simulink model "Crane_rigid"  (R2021b)
settings: Solver=ode15s  StartTime=0.0  StopTime=t_f  MaxStep=max_step_size  RelTol=1e-3
values from neighbouring files (symbols this model uses):
  a_d_full_y = circshift(a_d_full_x,floor(1/h))/2    [modify_tracking.m]
  cont_param_10 = in    [double_pendulum.m]    (also in optimize_10_SMC_single_first_explicit.m = cont_param_10_surrogateopt)
  cont_param_11 = in    [double_pendulum.m]    (also in optimize_11_SMC_single_first_implicit.m = cont_param_11_surrogateopt)
  cont_param_12 = in    [double_pendulum.m]    (also in optimize_12_SMC_single_last_explicit.m = cont_param_12_surrogateopt)
  cont_param_13 = in    [double_pendulum.m]    (also in optimize_13_SMC_single_last_implicit.m = cont_param_13_surrogateopt)
  cont_param_14 = in    [double_pendulum.m]    (also in optimize_14_SMC_double_explicit.m = cont_param_14_surrogateopt)
  cont_param_15 = in    [double_pendulum.m]    (also in optimize_15_SMC_double_implicit.m = cont_param_15_surrogateopt)
  cont_param_16 = in    [double_pendulum.m]
  cont_param_17 = in    [double_pendulum.m]
  cont_param_18 = in    [double_pendulum.m]
  cont_param_19 = in    [double_pendulum.m]
  cont_param_4 = in    [double_pendulum.m]
  cont_param_5 = in    [double_pendulum.m]
  cont_param_6 = in    [double_pendulum.m]
  cont_param_7 = in    [double_pendulum.m]
  cont_param_8 = in    [double_pendulum.m]
  cont_param_9 = in    [double_pendulum.m]
  h = 1e-5    (= 1e-05)    [Conference_paper.m]    (also in Latest.m)
  m = 10    [Conference_paper.m]    (also in Latest.m = 100; control_8_collocated_PD_tracking.m = load_mass+hook_mass+cable_mass_total)
  method_select = Method    [main_run.m]    (also in modify_tracking.m = 3)
  N = floor(t_f / h)    [control_2_zero_vibration.m]    (also in control_3_ZVD.m; modify_tracking.m = 3)
  s = c1*(x-xd)+c2*(v-vd)+c3*theta_dot_1+c4*theta_1    [control_10_SMC_single_first_explicit.m]    (also in control_11_SMC_single_first_implicit.m = c1*(x-xd)+c2*(v-vd)+c3*theta_dot+c4*theta; control_12_SMC_single_last_explicit.m = c1*(x-xd)+c2*(v-vd)+c3*theta_dot_2+c4*theta_2; control_13_SMC_single_last_implicit.m = c1*(x-xd)+c2*(v-vd)+c3*theta_dot+c4*theta; control_14_SMC_double_explicit.m = (v-vd)+lambda*(x-xd)+alpha*theta_1+beta*theta_2)
  sin_traj_w = 0.5    [modify_tracking.m]
  X = ex+lambda*sin(theta)    [control_16_PD_energy_first.m]    (also in control_17_PD_energy_last.m)
  Z = cont_param_8(4)    [control_8_collocated_PD_tracking.m]
undefined symbols (not defined in the file or in its folder): a_d_full_x, all_initial_sway, c_actuator, cable_length, cable_mass_total, cart_disturbance_amp, cart_mass, delay_time, first_link_sway, hook_mass, last_piece_length, load_disturbance_amp, number_of_pendulums, payload_mass, sat_const, sin_traj_A, t_f, total_mass, traj_number, unbalanced_factor, Y
libraries: nesl_utility x180, sm_lib x138, commchan3 x8
(part 3 of 3)

== system Crane_rigid/All pendulum/Angle sensor 2 ==
  Gain : Gain  Gain=-1
  Gain1 : Gain  Gain=-1
  PS-Simulink Converter{,1..7} (8 alike) : nesl_utility/PS-Simulink Converter  PhysicalDomain=network_engine_domain  SubClassName=ps_output  LeftPortType=input  RightPortType=output  PseudoPeriodic=off  Frequencies=[]  Unit=inherit  AffineConversion=off
      settings: SourceProductBaseCode=PW,SS
  Product : Product  Inputs=*/
  Product1 : Product  Inputs=*/
  Sin1 : Trigonometry  Operator=atan
  Sin2 : Trigonometry  Operator=atan
  Sum{,1..3} (4 alike) : Sum  Inputs=|+-
  Transform Sensor1 : sm_lib/Frames and Transforms/Transform Sensor  MeasurementFrame=World  SenseAngle=off  SenseAxis=off  SenseAngle1=off  SenseAngle2=off  SenseAngle3=off  SenseQ=off  SenseR=off  SenseOmegaX=off  SenseOmegaY=off  SenseOmegaZ=off  SenseOmega1=off  SenseOmega2=off  SenseOmega3=off  SenseQDot=off  SenseRDot=off  SenseAlphaX=off  SenseAlphaY=off  SenseAlphaZ=off  SenseAlpha1=off  SenseAlpha2=off  SenseAlpha3=off  SenseQDDot=off  SenseRDDot=off  SenseX=on  SenseY=on  SenseZ=on  SenseRad=off  SenseAzim=off  SenseDist=off  SenseInc=off  SenseXDot=off  SenseYDot=off  SenseZDot=off  SenseRadDot=off  SenseAzimDot=off  SenseDistDot=off  SenseIncDot=off  SenseXDDot=off  SenseYDDot=off  SenseZDDot=off  SenseRadDDot=off  SenseAzimDDot=off  SenseDistDDot=off  SenseIncDDot=off
  Transform Sensor2 : sm_lib/Frames and Transforms/Transform Sensor  MeasurementFrame=World  SenseAngle=off  SenseAxis=off  SenseAngle1=off  SenseAngle2=off  SenseAngle3=off  SenseQ=off  SenseR=off  SenseOmegaX=off  SenseOmegaY=off  SenseOmegaZ=off  SenseOmega1=off  SenseOmega2=off  SenseOmega3=off  SenseQDot=off  SenseRDot=off  SenseAlphaX=off  SenseAlphaY=off  SenseAlphaZ=off  SenseAlpha1=off  SenseAlpha2=off  SenseAlpha3=off  SenseQDDot=off  SenseRDDot=off  SenseX=on  SenseY=on  SenseZ=on  SenseRad=off  SenseAzim=off  SenseDist=off  SenseInc=off  SenseXDot=off  SenseYDot=off  SenseZDot=off  SenseRadDot=off  SenseAzimDot=off  SenseDistDot=off  SenseIncDot=off  SenseXDDot=off  SenseYDDot=off  SenseZDDot=off  SenseRadDDot=off  SenseAzimDDot=off  SenseDistDDot=off  SenseIncDDot=off
  World Frame : sm_lib/Frames and Transforms/World Frame
  Con1_up : PMIOPort  Side=Left
  Con2_down : PMIOPort  Port=2  Side=Left
  Angle_x : Outport
  Angle_y : Outport  Port=2
  wires:
  Sin1/1 -> Angle_y/1
  Sin2/1 -> Angle_x/1
  Sum/1 -> Gain/1
  Gain1/1 -> Product1/1
  Sum3/1 -> Product1/2
  Sum2/1 -> Gain1/1
  Product1/1 -> Sin1/1
  PS-Simulink Converter6/1 -> Sum3/1
  PS-Simulink Converter1/1 -> Sum/2
  PS-Simulink Converter5/1 -> Sum2/2
  PS-Simulink Converter4/1 -> Sum2/1
  PS-Simulink Converter7/1 -> Sum3/2
  Gain/1 -> Product/1
  PS-Simulink Converter3/1 -> Sum1/2
  PS-Simulink Converter2/1 -> Sum1/1
  Product/1 -> Sin2/1
  Sum1/1 -> Product/2
  PS-Simulink Converter/1 -> Sum/1
  connections:
  Con2_down/RConn1 -- Transform Sensor2/RConn1
  Transform Sensor1/RConn1 -- Con1_up/RConn1
  PS-Simulink Converter/LConn1 -- Transform Sensor1/RConn2
  Transform Sensor2/RConn2 -- PS-Simulink Converter1/LConn1
  PS-Simulink Converter4/LConn1 -- Transform Sensor1/RConn3
  PS-Simulink Converter5/LConn1 -- Transform Sensor2/RConn3
  PS-Simulink Converter2/LConn1 -- PS-Simulink Converter6/LConn1 -- Transform Sensor1/RConn4
  PS-Simulink Converter3/LConn1 -- PS-Simulink Converter7/LConn1 -- Transform Sensor2/RConn4
  Transform Sensor1/LConn1 -- Transform Sensor2/LConn1 -- World Frame/RConn1

== system Crane_rigid/All pendulum/Angle sensor 20 ==
  Gain : Gain  Gain=-1
  Gain1 : Gain  Gain=-1
  PS-Simulink Converter{,1..7} (8 alike) : nesl_utility/PS-Simulink Converter  PhysicalDomain=network_engine_domain  SubClassName=ps_output  LeftPortType=input  RightPortType=output  PseudoPeriodic=off  Frequencies=[]  Unit=inherit  AffineConversion=off
      settings: SourceProductBaseCode=PW,SS
  Product : Product  Inputs=*/
  Product1 : Product  Inputs=*/
  Sin1 : Trigonometry  Operator=atan
  Sin2 : Trigonometry  Operator=atan
  Sum{,1..3} (4 alike) : Sum  Inputs=|+-
  Transform Sensor1 : sm_lib/Frames and Transforms/Transform Sensor  MeasurementFrame=World  SenseAngle=off  SenseAxis=off  SenseAngle1=off  SenseAngle2=off  SenseAngle3=off  SenseQ=off  SenseR=off  SenseOmegaX=off  SenseOmegaY=off  SenseOmegaZ=off  SenseOmega1=off  SenseOmega2=off  SenseOmega3=off  SenseQDot=off  SenseRDot=off  SenseAlphaX=off  SenseAlphaY=off  SenseAlphaZ=off  SenseAlpha1=off  SenseAlpha2=off  SenseAlpha3=off  SenseQDDot=off  SenseRDDot=off  SenseX=on  SenseY=on  SenseZ=on  SenseRad=off  SenseAzim=off  SenseDist=off  SenseInc=off  SenseXDot=off  SenseYDot=off  SenseZDot=off  SenseRadDot=off  SenseAzimDot=off  SenseDistDot=off  SenseIncDot=off  SenseXDDot=off  SenseYDDot=off  SenseZDDot=off  SenseRadDDot=off  SenseAzimDDot=off  SenseDistDDot=off  SenseIncDDot=off
  Transform Sensor2 : sm_lib/Frames and Transforms/Transform Sensor  MeasurementFrame=World  SenseAngle=off  SenseAxis=off  SenseAngle1=off  SenseAngle2=off  SenseAngle3=off  SenseQ=off  SenseR=off  SenseOmegaX=off  SenseOmegaY=off  SenseOmegaZ=off  SenseOmega1=off  SenseOmega2=off  SenseOmega3=off  SenseQDot=off  SenseRDot=off  SenseAlphaX=off  SenseAlphaY=off  SenseAlphaZ=off  SenseAlpha1=off  SenseAlpha2=off  SenseAlpha3=off  SenseQDDot=off  SenseRDDot=off  SenseX=on  SenseY=on  SenseZ=on  SenseRad=off  SenseAzim=off  SenseDist=off  SenseInc=off  SenseXDot=off  SenseYDot=off  SenseZDot=off  SenseRadDot=off  SenseAzimDot=off  SenseDistDot=off  SenseIncDot=off  SenseXDDot=off  SenseYDDot=off  SenseZDDot=off  SenseRadDDot=off  SenseAzimDDot=off  SenseDistDDot=off  SenseIncDDot=off
  World Frame : sm_lib/Frames and Transforms/World Frame
  Con1_up : PMIOPort  Side=Left
  Con2_down : PMIOPort  Port=2  Side=Left
  Angle_x : Outport
  Angle_y : Outport  Port=2
  wires:
  Sin1/1 -> Angle_y/1
  Sin2/1 -> Angle_x/1
  Sum/1 -> Gain/1
  Gain1/1 -> Product1/1
  Sum3/1 -> Product1/2
  Sum2/1 -> Gain1/1
  Product1/1 -> Sin1/1
  PS-Simulink Converter6/1 -> Sum3/1
  PS-Simulink Converter1/1 -> Sum/2
  PS-Simulink Converter5/1 -> Sum2/2
  PS-Simulink Converter4/1 -> Sum2/1
  PS-Simulink Converter7/1 -> Sum3/2
  Gain/1 -> Product/1
  PS-Simulink Converter3/1 -> Sum1/2
  PS-Simulink Converter2/1 -> Sum1/1
  Product/1 -> Sin2/1
  Sum1/1 -> Product/2
  PS-Simulink Converter/1 -> Sum/1
  connections:
  Con2_down/RConn1 -- Transform Sensor2/RConn1
  Transform Sensor1/RConn1 -- Con1_up/RConn1
  PS-Simulink Converter/LConn1 -- Transform Sensor1/RConn2
  Transform Sensor2/RConn2 -- PS-Simulink Converter1/LConn1
  PS-Simulink Converter4/LConn1 -- Transform Sensor1/RConn3
  PS-Simulink Converter5/LConn1 -- Transform Sensor2/RConn3
  PS-Simulink Converter2/LConn1 -- PS-Simulink Converter6/LConn1 -- Transform Sensor1/RConn4
  PS-Simulink Converter3/LConn1 -- PS-Simulink Converter7/LConn1 -- Transform Sensor2/RConn4
  Transform Sensor1/LConn1 -- Transform Sensor2/LConn1 -- World Frame/RConn1

== system Crane_rigid/All pendulum/Angle sensor 21 ==
  Gain : Gain  Gain=-1
  Gain1 : Gain  Gain=-1
  PS-Simulink Converter{,1..7} (8 alike) : nesl_utility/PS-Simulink Converter  PhysicalDomain=network_engine_domain  SubClassName=ps_output  LeftPortType=input  RightPortType=output  PseudoPeriodic=off  Frequencies=[]  Unit=inherit  AffineConversion=off
      settings: SourceProductBaseCode=PW,SS
  Product : Product  Inputs=*/
  Product1 : Product  Inputs=*/
  Sin1 : Trigonometry  Operator=atan
  Sin2 : Trigonometry  Operator=atan
  Sum{,1..3} (4 alike) : Sum  Inputs=|+-
  Transform Sensor1 : sm_lib/Frames and Transforms/Transform Sensor  MeasurementFrame=World  SenseAngle=off  SenseAxis=off  SenseAngle1=off  SenseAngle2=off  SenseAngle3=off  SenseQ=off  SenseR=off  SenseOmegaX=off  SenseOmegaY=off  SenseOmegaZ=off  SenseOmega1=off  SenseOmega2=off  SenseOmega3=off  SenseQDot=off  SenseRDot=off  SenseAlphaX=off  SenseAlphaY=off  SenseAlphaZ=off  SenseAlpha1=off  SenseAlpha2=off  SenseAlpha3=off  SenseQDDot=off  SenseRDDot=off  SenseX=on  SenseY=on  SenseZ=on  SenseRad=off  SenseAzim=off  SenseDist=off  SenseInc=off  SenseXDot=off  SenseYDot=off  SenseZDot=off  SenseRadDot=off  SenseAzimDot=off  SenseDistDot=off  SenseIncDot=off  SenseXDDot=off  SenseYDDot=off  SenseZDDot=off  SenseRadDDot=off  SenseAzimDDot=off  SenseDistDDot=off  SenseIncDDot=off
  Transform Sensor2 : sm_lib/Frames and Transforms/Transform Sensor  MeasurementFrame=World  SenseAngle=off  SenseAxis=off  SenseAngle1=off  SenseAngle2=off  SenseAngle3=off  SenseQ=off  SenseR=off  SenseOmegaX=off  SenseOmegaY=off  SenseOmegaZ=off  SenseOmega1=off  SenseOmega2=off  SenseOmega3=off  SenseQDot=off  SenseRDot=off  SenseAlphaX=off  SenseAlphaY=off  SenseAlphaZ=off  SenseAlpha1=off  SenseAlpha2=off  SenseAlpha3=off  SenseQDDot=off  SenseRDDot=off  SenseX=on  SenseY=on  SenseZ=on  SenseRad=off  SenseAzim=off  SenseDist=off  SenseInc=off  SenseXDot=off  SenseYDot=off  SenseZDot=off  SenseRadDot=off  SenseAzimDot=off  SenseDistDot=off  SenseIncDot=off  SenseXDDot=off  SenseYDDot=off  SenseZDDot=off  SenseRadDDot=off  SenseAzimDDot=off  SenseDistDDot=off  SenseIncDDot=off
  World Frame : sm_lib/Frames and Transforms/World Frame
  Con1_up : PMIOPort  Side=Left
  Con2_down : PMIOPort  Port=2  Side=Left
  Angle_x : Outport
  Angle_y : Outport  Port=2
  wires:
  PS-Simulink Converter/1 -> Sum/1
  Sum1/1 -> Product/2
  Product/1 -> Sin2/1
  PS-Simulink Converter2/1 -> Sum1/1
  PS-Simulink Converter3/1 -> Sum1/2
  Gain/1 -> Product/1
  PS-Simulink Converter7/1 -> Sum3/2
  PS-Simulink Converter4/1 -> Sum2/1
  PS-Simulink Converter5/1 -> Sum2/2
  PS-Simulink Converter1/1 -> Sum/2
  PS-Simulink Converter6/1 -> Sum3/1
  Product1/1 -> Sin1/1
  Sum2/1 -> Gain1/1
  Sum3/1 -> Product1/2
  Gain1/1 -> Product1/1
  Sum/1 -> Gain/1
  Sin2/1 -> Angle_x/1
  Sin1/1 -> Angle_y/1
  connections:
  World Frame/RConn1 -- Transform Sensor2/LConn1 -- Transform Sensor1/LConn1
  Transform Sensor2/RConn4 -- PS-Simulink Converter7/LConn1 -- PS-Simulink Converter3/LConn1
  Transform Sensor1/RConn4 -- PS-Simulink Converter6/LConn1 -- PS-Simulink Converter2/LConn1
  PS-Simulink Converter5/LConn1 -- Transform Sensor2/RConn3
  PS-Simulink Converter4/LConn1 -- Transform Sensor1/RConn3
  Transform Sensor2/RConn2 -- PS-Simulink Converter1/LConn1
  PS-Simulink Converter/LConn1 -- Transform Sensor1/RConn2
  Transform Sensor1/RConn1 -- Con1_up/RConn1
  Con2_down/RConn1 -- Transform Sensor2/RConn1

== system Crane_rigid/All pendulum/Angle sensor 3 ==
  Gain : Gain  Gain=-1
  Gain1 : Gain  Gain=-1
  PS-Simulink Converter{,1..7} (8 alike) : nesl_utility/PS-Simulink Converter  PhysicalDomain=network_engine_domain  SubClassName=ps_output  LeftPortType=input  RightPortType=output  PseudoPeriodic=off  Frequencies=[]  Unit=inherit  AffineConversion=off
      settings: SourceProductBaseCode=PW,SS
  Product : Product  Inputs=*/
  Product1 : Product  Inputs=*/
  Sin1 : Trigonometry  Operator=atan
  Sin2 : Trigonometry  Operator=atan
  Sum{,1..3} (4 alike) : Sum  Inputs=|+-
  Transform Sensor1 : sm_lib/Frames and Transforms/Transform Sensor  MeasurementFrame=World  SenseAngle=off  SenseAxis=off  SenseAngle1=off  SenseAngle2=off  SenseAngle3=off  SenseQ=off  SenseR=off  SenseOmegaX=off  SenseOmegaY=off  SenseOmegaZ=off  SenseOmega1=off  SenseOmega2=off  SenseOmega3=off  SenseQDot=off  SenseRDot=off  SenseAlphaX=off  SenseAlphaY=off  SenseAlphaZ=off  SenseAlpha1=off  SenseAlpha2=off  SenseAlpha3=off  SenseQDDot=off  SenseRDDot=off  SenseX=on  SenseY=on  SenseZ=on  SenseRad=off  SenseAzim=off  SenseDist=off  SenseInc=off  SenseXDot=off  SenseYDot=off  SenseZDot=off  SenseRadDot=off  SenseAzimDot=off  SenseDistDot=off  SenseIncDot=off  SenseXDDot=off  SenseYDDot=off  SenseZDDot=off  SenseRadDDot=off  SenseAzimDDot=off  SenseDistDDot=off  SenseIncDDot=off
  Transform Sensor2 : sm_lib/Frames and Transforms/Transform Sensor  MeasurementFrame=World  SenseAngle=off  SenseAxis=off  SenseAngle1=off  SenseAngle2=off  SenseAngle3=off  SenseQ=off  SenseR=off  SenseOmegaX=off  SenseOmegaY=off  SenseOmegaZ=off  SenseOmega1=off  SenseOmega2=off  SenseOmega3=off  SenseQDot=off  SenseRDot=off  SenseAlphaX=off  SenseAlphaY=off  SenseAlphaZ=off  SenseAlpha1=off  SenseAlpha2=off  SenseAlpha3=off  SenseQDDot=off  SenseRDDot=off  SenseX=on  SenseY=on  SenseZ=on  SenseRad=off  SenseAzim=off  SenseDist=off  SenseInc=off  SenseXDot=off  SenseYDot=off  SenseZDot=off  SenseRadDot=off  SenseAzimDot=off  SenseDistDot=off  SenseIncDot=off  SenseXDDot=off  SenseYDDot=off  SenseZDDot=off  SenseRadDDot=off  SenseAzimDDot=off  SenseDistDDot=off  SenseIncDDot=off
  World Frame : sm_lib/Frames and Transforms/World Frame
  Con1_up : PMIOPort  Side=Left
  Con2_down : PMIOPort  Port=2  Side=Left
  Angle_x : Outport
  Angle_y : Outport  Port=2
  wires:
  Sin1/1 -> Angle_y/1
  Sin2/1 -> Angle_x/1
  Sum/1 -> Gain/1
  Gain1/1 -> Product1/1
  Sum3/1 -> Product1/2
  Sum2/1 -> Gain1/1
  Product1/1 -> Sin1/1
  PS-Simulink Converter6/1 -> Sum3/1
  PS-Simulink Converter1/1 -> Sum/2
  PS-Simulink Converter5/1 -> Sum2/2
  PS-Simulink Converter4/1 -> Sum2/1
  PS-Simulink Converter7/1 -> Sum3/2
  Gain/1 -> Product/1
  PS-Simulink Converter3/1 -> Sum1/2
  PS-Simulink Converter2/1 -> Sum1/1
  Product/1 -> Sin2/1
  Sum1/1 -> Product/2
  PS-Simulink Converter/1 -> Sum/1
  connections:
  Con2_down/RConn1 -- Transform Sensor2/RConn1
  Transform Sensor1/RConn1 -- Con1_up/RConn1
  PS-Simulink Converter/LConn1 -- Transform Sensor1/RConn2
  Transform Sensor2/RConn2 -- PS-Simulink Converter1/LConn1
  PS-Simulink Converter4/LConn1 -- Transform Sensor1/RConn3
  PS-Simulink Converter5/LConn1 -- Transform Sensor2/RConn3
  PS-Simulink Converter2/LConn1 -- PS-Simulink Converter6/LConn1 -- Transform Sensor1/RConn4
  PS-Simulink Converter3/LConn1 -- PS-Simulink Converter7/LConn1 -- Transform Sensor2/RConn4
  Transform Sensor1/LConn1 -- Transform Sensor2/LConn1 -- World Frame/RConn1

== system Crane_rigid/All pendulum/Angle sensor 4 ==
  Gain : Gain  Gain=-1
  Gain1 : Gain  Gain=-1
  PS-Simulink Converter{,1..7} (8 alike) : nesl_utility/PS-Simulink Converter  PhysicalDomain=network_engine_domain  SubClassName=ps_output  LeftPortType=input  RightPortType=output  PseudoPeriodic=off  Frequencies=[]  Unit=inherit  AffineConversion=off
      settings: SourceProductBaseCode=PW,SS
  Product : Product  Inputs=*/
  Product1 : Product  Inputs=*/
  Sin1 : Trigonometry  Operator=atan
  Sin2 : Trigonometry  Operator=atan
  Sum{,1..3} (4 alike) : Sum  Inputs=|+-
  Transform Sensor1 : sm_lib/Frames and Transforms/Transform Sensor  MeasurementFrame=World  SenseAngle=off  SenseAxis=off  SenseAngle1=off  SenseAngle2=off  SenseAngle3=off  SenseQ=off  SenseR=off  SenseOmegaX=off  SenseOmegaY=off  SenseOmegaZ=off  SenseOmega1=off  SenseOmega2=off  SenseOmega3=off  SenseQDot=off  SenseRDot=off  SenseAlphaX=off  SenseAlphaY=off  SenseAlphaZ=off  SenseAlpha1=off  SenseAlpha2=off  SenseAlpha3=off  SenseQDDot=off  SenseRDDot=off  SenseX=on  SenseY=on  SenseZ=on  SenseRad=off  SenseAzim=off  SenseDist=off  SenseInc=off  SenseXDot=off  SenseYDot=off  SenseZDot=off  SenseRadDot=off  SenseAzimDot=off  SenseDistDot=off  SenseIncDot=off  SenseXDDot=off  SenseYDDot=off  SenseZDDot=off  SenseRadDDot=off  SenseAzimDDot=off  SenseDistDDot=off  SenseIncDDot=off
  Transform Sensor2 : sm_lib/Frames and Transforms/Transform Sensor  MeasurementFrame=World  SenseAngle=off  SenseAxis=off  SenseAngle1=off  SenseAngle2=off  SenseAngle3=off  SenseQ=off  SenseR=off  SenseOmegaX=off  SenseOmegaY=off  SenseOmegaZ=off  SenseOmega1=off  SenseOmega2=off  SenseOmega3=off  SenseQDot=off  SenseRDot=off  SenseAlphaX=off  SenseAlphaY=off  SenseAlphaZ=off  SenseAlpha1=off  SenseAlpha2=off  SenseAlpha3=off  SenseQDDot=off  SenseRDDot=off  SenseX=on  SenseY=on  SenseZ=on  SenseRad=off  SenseAzim=off  SenseDist=off  SenseInc=off  SenseXDot=off  SenseYDot=off  SenseZDot=off  SenseRadDot=off  SenseAzimDot=off  SenseDistDot=off  SenseIncDot=off  SenseXDDot=off  SenseYDDot=off  SenseZDDot=off  SenseRadDDot=off  SenseAzimDDot=off  SenseDistDDot=off  SenseIncDDot=off
  World Frame : sm_lib/Frames and Transforms/World Frame
  Con1_up : PMIOPort  Side=Left
  Con2_down : PMIOPort  Port=2  Side=Left
  Angle_x : Outport
  Angle_y : Outport  Port=2
  wires:
  Sin1/1 -> Angle_y/1
  Sin2/1 -> Angle_x/1
  Sum/1 -> Gain/1
  Gain1/1 -> Product1/1
  Sum3/1 -> Product1/2
  Sum2/1 -> Gain1/1
  Product1/1 -> Sin1/1
  PS-Simulink Converter6/1 -> Sum3/1
  PS-Simulink Converter1/1 -> Sum/2
  PS-Simulink Converter5/1 -> Sum2/2
  PS-Simulink Converter4/1 -> Sum2/1
  PS-Simulink Converter7/1 -> Sum3/2
  Gain/1 -> Product/1
  PS-Simulink Converter3/1 -> Sum1/2
  PS-Simulink Converter2/1 -> Sum1/1
  Product/1 -> Sin2/1
  Sum1/1 -> Product/2
  PS-Simulink Converter/1 -> Sum/1
  connections:
  Con2_down/RConn1 -- Transform Sensor2/RConn1
  Transform Sensor1/RConn1 -- Con1_up/RConn1
  PS-Simulink Converter/LConn1 -- Transform Sensor1/RConn2
  Transform Sensor2/RConn2 -- PS-Simulink Converter1/LConn1
  PS-Simulink Converter4/LConn1 -- Transform Sensor1/RConn3
  PS-Simulink Converter5/LConn1 -- Transform Sensor2/RConn3
  PS-Simulink Converter2/LConn1 -- PS-Simulink Converter6/LConn1 -- Transform Sensor1/RConn4
  PS-Simulink Converter3/LConn1 -- PS-Simulink Converter7/LConn1 -- Transform Sensor2/RConn4
  Transform Sensor1/LConn1 -- Transform Sensor2/LConn1 -- World Frame/RConn1

== system Crane_rigid/All pendulum/Angle sensor 5 ==
  Gain : Gain  Gain=-1
  Gain1 : Gain  Gain=-1
  PS-Simulink Converter{,1..7} (8 alike) : nesl_utility/PS-Simulink Converter  PhysicalDomain=network_engine_domain  SubClassName=ps_output  LeftPortType=input  RightPortType=output  PseudoPeriodic=off  Frequencies=[]  Unit=inherit  AffineConversion=off
      settings: SourceProductBaseCode=PW,SS
  Product : Product  Inputs=*/
  Product1 : Product  Inputs=*/
  Sin1 : Trigonometry  Operator=atan
  Sin2 : Trigonometry  Operator=atan
  Sum{,1..3} (4 alike) : Sum  Inputs=|+-
  Transform Sensor1 : sm_lib/Frames and Transforms/Transform Sensor  MeasurementFrame=World  SenseAngle=off  SenseAxis=off  SenseAngle1=off  SenseAngle2=off  SenseAngle3=off  SenseQ=off  SenseR=off  SenseOmegaX=off  SenseOmegaY=off  SenseOmegaZ=off  SenseOmega1=off  SenseOmega2=off  SenseOmega3=off  SenseQDot=off  SenseRDot=off  SenseAlphaX=off  SenseAlphaY=off  SenseAlphaZ=off  SenseAlpha1=off  SenseAlpha2=off  SenseAlpha3=off  SenseQDDot=off  SenseRDDot=off  SenseX=on  SenseY=on  SenseZ=on  SenseRad=off  SenseAzim=off  SenseDist=off  SenseInc=off  SenseXDot=off  SenseYDot=off  SenseZDot=off  SenseRadDot=off  SenseAzimDot=off  SenseDistDot=off  SenseIncDot=off  SenseXDDot=off  SenseYDDot=off  SenseZDDot=off  SenseRadDDot=off  SenseAzimDDot=off  SenseDistDDot=off  SenseIncDDot=off
  Transform Sensor2 : sm_lib/Frames and Transforms/Transform Sensor  MeasurementFrame=World  SenseAngle=off  SenseAxis=off  SenseAngle1=off  SenseAngle2=off  SenseAngle3=off  SenseQ=off  SenseR=off  SenseOmegaX=off  SenseOmegaY=off  SenseOmegaZ=off  SenseOmega1=off  SenseOmega2=off  SenseOmega3=off  SenseQDot=off  SenseRDot=off  SenseAlphaX=off  SenseAlphaY=off  SenseAlphaZ=off  SenseAlpha1=off  SenseAlpha2=off  SenseAlpha3=off  SenseQDDot=off  SenseRDDot=off  SenseX=on  SenseY=on  SenseZ=on  SenseRad=off  SenseAzim=off  SenseDist=off  SenseInc=off  SenseXDot=off  SenseYDot=off  SenseZDot=off  SenseRadDot=off  SenseAzimDot=off  SenseDistDot=off  SenseIncDot=off  SenseXDDot=off  SenseYDDot=off  SenseZDDot=off  SenseRadDDot=off  SenseAzimDDot=off  SenseDistDDot=off  SenseIncDDot=off
  World Frame : sm_lib/Frames and Transforms/World Frame
  Con1_up : PMIOPort  Side=Left
  Con2_down : PMIOPort  Port=2  Side=Left
  Angle_x : Outport
  Angle_y : Outport  Port=2
  wires:
  PS-Simulink Converter/1 -> Sum/1
  Sum1/1 -> Product/2
  Product/1 -> Sin2/1
  PS-Simulink Converter2/1 -> Sum1/1
  PS-Simulink Converter3/1 -> Sum1/2
  Gain/1 -> Product/1
  PS-Simulink Converter7/1 -> Sum3/2
  PS-Simulink Converter4/1 -> Sum2/1
  PS-Simulink Converter5/1 -> Sum2/2
  PS-Simulink Converter1/1 -> Sum/2
  PS-Simulink Converter6/1 -> Sum3/1
  Product1/1 -> Sin1/1
  Sum2/1 -> Gain1/1
  Sum3/1 -> Product1/2
  Gain1/1 -> Product1/1
  Sum/1 -> Gain/1
  Sin2/1 -> Angle_x/1
  Sin1/1 -> Angle_y/1
  connections:
  World Frame/RConn1 -- Transform Sensor2/LConn1 -- Transform Sensor1/LConn1
  Transform Sensor2/RConn4 -- PS-Simulink Converter7/LConn1 -- PS-Simulink Converter3/LConn1
  Transform Sensor1/RConn4 -- PS-Simulink Converter6/LConn1 -- PS-Simulink Converter2/LConn1
  PS-Simulink Converter5/LConn1 -- Transform Sensor2/RConn3
  PS-Simulink Converter4/LConn1 -- Transform Sensor1/RConn3
  Transform Sensor2/RConn2 -- PS-Simulink Converter1/LConn1
  PS-Simulink Converter/LConn1 -- Transform Sensor1/RConn2
  Transform Sensor1/RConn1 -- Con1_up/RConn1
  Con2_down/RConn1 -- Transform Sensor2/RConn1

== system Crane_rigid/All pendulum/Angle sensor 6 ==
  Gain : Gain  Gain=-1
  Gain1 : Gain  Gain=-1
  PS-Simulink Converter{,1..7} (8 alike) : nesl_utility/PS-Simulink Converter  PhysicalDomain=network_engine_domain  SubClassName=ps_output  LeftPortType=input  RightPortType=output  PseudoPeriodic=off  Frequencies=[]  Unit=inherit  AffineConversion=off
      settings: SourceProductBaseCode=PW,SS
  Product : Product  Inputs=*/
  Product1 : Product  Inputs=*/
  Sin1 : Trigonometry  Operator=atan
  Sin2 : Trigonometry  Operator=atan
  Sum{,1..3} (4 alike) : Sum  Inputs=|+-
  Transform Sensor1 : sm_lib/Frames and Transforms/Transform Sensor  MeasurementFrame=World  SenseAngle=off  SenseAxis=off  SenseAngle1=off  SenseAngle2=off  SenseAngle3=off  SenseQ=off  SenseR=off  SenseOmegaX=off  SenseOmegaY=off  SenseOmegaZ=off  SenseOmega1=off  SenseOmega2=off  SenseOmega3=off  SenseQDot=off  SenseRDot=off  SenseAlphaX=off  SenseAlphaY=off  SenseAlphaZ=off  SenseAlpha1=off  SenseAlpha2=off  SenseAlpha3=off  SenseQDDot=off  SenseRDDot=off  SenseX=on  SenseY=on  SenseZ=on  SenseRad=off  SenseAzim=off  SenseDist=off  SenseInc=off  SenseXDot=off  SenseYDot=off  SenseZDot=off  SenseRadDot=off  SenseAzimDot=off  SenseDistDot=off  SenseIncDot=off  SenseXDDot=off  SenseYDDot=off  SenseZDDot=off  SenseRadDDot=off  SenseAzimDDot=off  SenseDistDDot=off  SenseIncDDot=off
  Transform Sensor2 : sm_lib/Frames and Transforms/Transform Sensor  MeasurementFrame=World  SenseAngle=off  SenseAxis=off  SenseAngle1=off  SenseAngle2=off  SenseAngle3=off  SenseQ=off  SenseR=off  SenseOmegaX=off  SenseOmegaY=off  SenseOmegaZ=off  SenseOmega1=off  SenseOmega2=off  SenseOmega3=off  SenseQDot=off  SenseRDot=off  SenseAlphaX=off  SenseAlphaY=off  SenseAlphaZ=off  SenseAlpha1=off  SenseAlpha2=off  SenseAlpha3=off  SenseQDDot=off  SenseRDDot=off  SenseX=on  SenseY=on  SenseZ=on  SenseRad=off  SenseAzim=off  SenseDist=off  SenseInc=off  SenseXDot=off  SenseYDot=off  SenseZDot=off  SenseRadDot=off  SenseAzimDot=off  SenseDistDot=off  SenseIncDot=off  SenseXDDot=off  SenseYDDot=off  SenseZDDot=off  SenseRadDDot=off  SenseAzimDDot=off  SenseDistDDot=off  SenseIncDDot=off
  World Frame : sm_lib/Frames and Transforms/World Frame
  Con1_up : PMIOPort  Side=Left
  Con2_down : PMIOPort  Port=2  Side=Left
  Angle_x : Outport
  Angle_y : Outport  Port=2
  wires:
  Sin1/1 -> Angle_y/1
  Sin2/1 -> Angle_x/1
  Sum/1 -> Gain/1
  Gain1/1 -> Product1/1
  Sum3/1 -> Product1/2
  Sum2/1 -> Gain1/1
  Product1/1 -> Sin1/1
  PS-Simulink Converter6/1 -> Sum3/1
  PS-Simulink Converter1/1 -> Sum/2
  PS-Simulink Converter5/1 -> Sum2/2
  PS-Simulink Converter4/1 -> Sum2/1
  PS-Simulink Converter7/1 -> Sum3/2
  Gain/1 -> Product/1
  PS-Simulink Converter3/1 -> Sum1/2
  PS-Simulink Converter2/1 -> Sum1/1
  Product/1 -> Sin2/1
  Sum1/1 -> Product/2
  PS-Simulink Converter/1 -> Sum/1
  connections:
  Con2_down/RConn1 -- Transform Sensor2/RConn1
  Transform Sensor1/RConn1 -- Con1_up/RConn1
  PS-Simulink Converter/LConn1 -- Transform Sensor1/RConn2
  Transform Sensor2/RConn2 -- PS-Simulink Converter1/LConn1
  PS-Simulink Converter4/LConn1 -- Transform Sensor1/RConn3
  PS-Simulink Converter5/LConn1 -- Transform Sensor2/RConn3
  PS-Simulink Converter2/LConn1 -- PS-Simulink Converter6/LConn1 -- Transform Sensor1/RConn4
  PS-Simulink Converter3/LConn1 -- PS-Simulink Converter7/LConn1 -- Transform Sensor2/RConn4
  Transform Sensor1/LConn1 -- Transform Sensor2/LConn1 -- World Frame/RConn1

== system Crane_rigid/All pendulum/Angle sensor 7 ==
  Gain : Gain  Gain=-1
  Gain1 : Gain  Gain=-1
  PS-Simulink Converter{,1..7} (8 alike) : nesl_utility/PS-Simulink Converter  PhysicalDomain=network_engine_domain  SubClassName=ps_output  LeftPortType=input  RightPortType=output  PseudoPeriodic=off  Frequencies=[]  Unit=inherit  AffineConversion=off
      settings: SourceProductBaseCode=PW,SS
  Product : Product  Inputs=*/
  Product1 : Product  Inputs=*/
  Sin1 : Trigonometry  Operator=atan
  Sin2 : Trigonometry  Operator=atan
  Sum{,1..3} (4 alike) : Sum  Inputs=|+-
  Transform Sensor1 : sm_lib/Frames and Transforms/Transform Sensor  MeasurementFrame=World  SenseAngle=off  SenseAxis=off  SenseAngle1=off  SenseAngle2=off  SenseAngle3=off  SenseQ=off  SenseR=off  SenseOmegaX=off  SenseOmegaY=off  SenseOmegaZ=off  SenseOmega1=off  SenseOmega2=off  SenseOmega3=off  SenseQDot=off  SenseRDot=off  SenseAlphaX=off  SenseAlphaY=off  SenseAlphaZ=off  SenseAlpha1=off  SenseAlpha2=off  SenseAlpha3=off  SenseQDDot=off  SenseRDDot=off  SenseX=on  SenseY=on  SenseZ=on  SenseRad=off  SenseAzim=off  SenseDist=off  SenseInc=off  SenseXDot=off  SenseYDot=off  SenseZDot=off  SenseRadDot=off  SenseAzimDot=off  SenseDistDot=off  SenseIncDot=off  SenseXDDot=off  SenseYDDot=off  SenseZDDot=off  SenseRadDDot=off  SenseAzimDDot=off  SenseDistDDot=off  SenseIncDDot=off
  Transform Sensor2 : sm_lib/Frames and Transforms/Transform Sensor  MeasurementFrame=World  SenseAngle=off  SenseAxis=off  SenseAngle1=off  SenseAngle2=off  SenseAngle3=off  SenseQ=off  SenseR=off  SenseOmegaX=off  SenseOmegaY=off  SenseOmegaZ=off  SenseOmega1=off  SenseOmega2=off  SenseOmega3=off  SenseQDot=off  SenseRDot=off  SenseAlphaX=off  SenseAlphaY=off  SenseAlphaZ=off  SenseAlpha1=off  SenseAlpha2=off  SenseAlpha3=off  SenseQDDot=off  SenseRDDot=off  SenseX=on  SenseY=on  SenseZ=on  SenseRad=off  SenseAzim=off  SenseDist=off  SenseInc=off  SenseXDot=off  SenseYDot=off  SenseZDot=off  SenseRadDot=off  SenseAzimDot=off  SenseDistDot=off  SenseIncDot=off  SenseXDDot=off  SenseYDDot=off  SenseZDDot=off  SenseRadDDot=off  SenseAzimDDot=off  SenseDistDDot=off  SenseIncDDot=off
  World Frame : sm_lib/Frames and Transforms/World Frame
  Con1_up : PMIOPort  Side=Left
  Con2_down : PMIOPort  Port=2  Side=Left
  Angle_x : Outport
  Angle_y : Outport  Port=2
  wires:
  PS-Simulink Converter/1 -> Sum/1
  Sum1/1 -> Product/2
  Product/1 -> Sin2/1
  PS-Simulink Converter2/1 -> Sum1/1
  PS-Simulink Converter3/1 -> Sum1/2
  Gain/1 -> Product/1
  PS-Simulink Converter7/1 -> Sum3/2
  PS-Simulink Converter4/1 -> Sum2/1
  PS-Simulink Converter5/1 -> Sum2/2
  PS-Simulink Converter1/1 -> Sum/2
  PS-Simulink Converter6/1 -> Sum3/1
  Product1/1 -> Sin1/1
  Sum2/1 -> Gain1/1
  Sum3/1 -> Product1/2
  Gain1/1 -> Product1/1
  Sum/1 -> Gain/1
  Sin2/1 -> Angle_x/1
  Sin1/1 -> Angle_y/1
  connections:
  World Frame/RConn1 -- Transform Sensor2/LConn1 -- Transform Sensor1/LConn1
  Transform Sensor2/RConn4 -- PS-Simulink Converter7/LConn1 -- PS-Simulink Converter3/LConn1
  Transform Sensor1/RConn4 -- PS-Simulink Converter6/LConn1 -- PS-Simulink Converter2/LConn1
  PS-Simulink Converter5/LConn1 -- Transform Sensor2/RConn3
  PS-Simulink Converter4/LConn1 -- Transform Sensor1/RConn3
  Transform Sensor2/RConn2 -- PS-Simulink Converter1/LConn1
  PS-Simulink Converter/LConn1 -- Transform Sensor1/RConn2
  Transform Sensor1/RConn1 -- Con1_up/RConn1
  Con2_down/RConn1 -- Transform Sensor2/RConn1

== system Crane_rigid/All pendulum/Angle sensor 8 ==
  Gain : Gain  Gain=-1
  Gain1 : Gain  Gain=-1
  PS-Simulink Converter{,1..7} (8 alike) : nesl_utility/PS-Simulink Converter  PhysicalDomain=network_engine_domain  SubClassName=ps_output  LeftPortType=input  RightPortType=output  PseudoPeriodic=off  Frequencies=[]  Unit=inherit  AffineConversion=off
      settings: SourceProductBaseCode=PW,SS
  Product : Product  Inputs=*/
  Product1 : Product  Inputs=*/
  Sin1 : Trigonometry  Operator=atan
  Sin2 : Trigonometry  Operator=atan
  Sum{,1..3} (4 alike) : Sum  Inputs=|+-
  Transform Sensor1 : sm_lib/Frames and Transforms/Transform Sensor  MeasurementFrame=World  SenseAngle=off  SenseAxis=off  SenseAngle1=off  SenseAngle2=off  SenseAngle3=off  SenseQ=off  SenseR=off  SenseOmegaX=off  SenseOmegaY=off  SenseOmegaZ=off  SenseOmega1=off  SenseOmega2=off  SenseOmega3=off  SenseQDot=off  SenseRDot=off  SenseAlphaX=off  SenseAlphaY=off  SenseAlphaZ=off  SenseAlpha1=off  SenseAlpha2=off  SenseAlpha3=off  SenseQDDot=off  SenseRDDot=off  SenseX=on  SenseY=on  SenseZ=on  SenseRad=off  SenseAzim=off  SenseDist=off  SenseInc=off  SenseXDot=off  SenseYDot=off  SenseZDot=off  SenseRadDot=off  SenseAzimDot=off  SenseDistDot=off  SenseIncDot=off  SenseXDDot=off  SenseYDDot=off  SenseZDDot=off  SenseRadDDot=off  SenseAzimDDot=off  SenseDistDDot=off  SenseIncDDot=off
  Transform Sensor2 : sm_lib/Frames and Transforms/Transform Sensor  MeasurementFrame=World  SenseAngle=off  SenseAxis=off  SenseAngle1=off  SenseAngle2=off  SenseAngle3=off  SenseQ=off  SenseR=off  SenseOmegaX=off  SenseOmegaY=off  SenseOmegaZ=off  SenseOmega1=off  SenseOmega2=off  SenseOmega3=off  SenseQDot=off  SenseRDot=off  SenseAlphaX=off  SenseAlphaY=off  SenseAlphaZ=off  SenseAlpha1=off  SenseAlpha2=off  SenseAlpha3=off  SenseQDDot=off  SenseRDDot=off  SenseX=on  SenseY=on  SenseZ=on  SenseRad=off  SenseAzim=off  SenseDist=off  SenseInc=off  SenseXDot=off  SenseYDot=off  SenseZDot=off  SenseRadDot=off  SenseAzimDot=off  SenseDistDot=off  SenseIncDot=off  SenseXDDot=off  SenseYDDot=off  SenseZDDot=off  SenseRadDDot=off  SenseAzimDDot=off  SenseDistDDot=off  SenseIncDDot=off
  World Frame : sm_lib/Frames and Transforms/World Frame
  Con1_up : PMIOPort  Side=Left
  Con2_down : PMIOPort  Port=2  Side=Left
  Angle_x : Outport
  Angle_y : Outport  Port=2
  wires:
  Sin1/1 -> Angle_y/1
  Sin2/1 -> Angle_x/1
  Sum/1 -> Gain/1
  Gain1/1 -> Product1/1
  Sum3/1 -> Product1/2
  Sum2/1 -> Gain1/1
  Product1/1 -> Sin1/1
  PS-Simulink Converter6/1 -> Sum3/1
  PS-Simulink Converter1/1 -> Sum/2
  PS-Simulink Converter5/1 -> Sum2/2
  PS-Simulink Converter4/1 -> Sum2/1
  PS-Simulink Converter7/1 -> Sum3/2
  Gain/1 -> Product/1
  PS-Simulink Converter3/1 -> Sum1/2
  PS-Simulink Converter2/1 -> Sum1/1
  Product/1 -> Sin2/1
  Sum1/1 -> Product/2
  PS-Simulink Converter/1 -> Sum/1
  connections:
  Con2_down/RConn1 -- Transform Sensor2/RConn1
  Transform Sensor1/RConn1 -- Con1_up/RConn1
  PS-Simulink Converter/LConn1 -- Transform Sensor1/RConn2
  Transform Sensor2/RConn2 -- PS-Simulink Converter1/LConn1
  PS-Simulink Converter4/LConn1 -- Transform Sensor1/RConn3
  PS-Simulink Converter5/LConn1 -- Transform Sensor2/RConn3
  PS-Simulink Converter2/LConn1 -- PS-Simulink Converter6/LConn1 -- Transform Sensor1/RConn4
  PS-Simulink Converter3/LConn1 -- PS-Simulink Converter7/LConn1 -- Transform Sensor2/RConn4
  Transform Sensor1/LConn1 -- Transform Sensor2/LConn1 -- World Frame/RConn1

== system Crane_rigid/All pendulum/Angle sensor 9 ==
  Gain : Gain  Gain=-1
  Gain1 : Gain  Gain=-1
  PS-Simulink Converter{,1..7} (8 alike) : nesl_utility/PS-Simulink Converter  PhysicalDomain=network_engine_domain  SubClassName=ps_output  LeftPortType=input  RightPortType=output  PseudoPeriodic=off  Frequencies=[]  Unit=inherit  AffineConversion=off
      settings: SourceProductBaseCode=PW,SS
  Product : Product  Inputs=*/
  Product1 : Product  Inputs=*/
  Sin1 : Trigonometry  Operator=atan
  Sin2 : Trigonometry  Operator=atan
  Sum{,1..3} (4 alike) : Sum  Inputs=|+-
  Transform Sensor1 : sm_lib/Frames and Transforms/Transform Sensor  MeasurementFrame=World  SenseAngle=off  SenseAxis=off  SenseAngle1=off  SenseAngle2=off  SenseAngle3=off  SenseQ=off  SenseR=off  SenseOmegaX=off  SenseOmegaY=off  SenseOmegaZ=off  SenseOmega1=off  SenseOmega2=off  SenseOmega3=off  SenseQDot=off  SenseRDot=off  SenseAlphaX=off  SenseAlphaY=off  SenseAlphaZ=off  SenseAlpha1=off  SenseAlpha2=off  SenseAlpha3=off  SenseQDDot=off  SenseRDDot=off  SenseX=on  SenseY=on  SenseZ=on  SenseRad=off  SenseAzim=off  SenseDist=off  SenseInc=off  SenseXDot=off  SenseYDot=off  SenseZDot=off  SenseRadDot=off  SenseAzimDot=off  SenseDistDot=off  SenseIncDot=off  SenseXDDot=off  SenseYDDot=off  SenseZDDot=off  SenseRadDDot=off  SenseAzimDDot=off  SenseDistDDot=off  SenseIncDDot=off
  Transform Sensor2 : sm_lib/Frames and Transforms/Transform Sensor  MeasurementFrame=World  SenseAngle=off  SenseAxis=off  SenseAngle1=off  SenseAngle2=off  SenseAngle3=off  SenseQ=off  SenseR=off  SenseOmegaX=off  SenseOmegaY=off  SenseOmegaZ=off  SenseOmega1=off  SenseOmega2=off  SenseOmega3=off  SenseQDot=off  SenseRDot=off  SenseAlphaX=off  SenseAlphaY=off  SenseAlphaZ=off  SenseAlpha1=off  SenseAlpha2=off  SenseAlpha3=off  SenseQDDot=off  SenseRDDot=off  SenseX=on  SenseY=on  SenseZ=on  SenseRad=off  SenseAzim=off  SenseDist=off  SenseInc=off  SenseXDot=off  SenseYDot=off  SenseZDot=off  SenseRadDot=off  SenseAzimDot=off  SenseDistDot=off  SenseIncDot=off  SenseXDDot=off  SenseYDDot=off  SenseZDDot=off  SenseRadDDot=off  SenseAzimDDot=off  SenseDistDDot=off  SenseIncDDot=off
  World Frame : sm_lib/Frames and Transforms/World Frame
  Con1_up : PMIOPort  Side=Left
  Con2_down : PMIOPort  Port=2  Side=Left
  Angle_x : Outport
  Angle_y : Outport  Port=2
  wires:
  PS-Simulink Converter/1 -> Sum/1
  Sum1/1 -> Product/2
  Product/1 -> Sin2/1
  PS-Simulink Converter2/1 -> Sum1/1
  PS-Simulink Converter3/1 -> Sum1/2
  Gain/1 -> Product/1
  PS-Simulink Converter7/1 -> Sum3/2
  PS-Simulink Converter4/1 -> Sum2/1
  PS-Simulink Converter5/1 -> Sum2/2
  PS-Simulink Converter1/1 -> Sum/2
  PS-Simulink Converter6/1 -> Sum3/1
  Product1/1 -> Sin1/1
  Sum2/1 -> Gain1/1
  Sum3/1 -> Product1/2
  Gain1/1 -> Product1/1
  Sum/1 -> Gain/1
  Sin2/1 -> Angle_x/1
  Sin1/1 -> Angle_y/1
  connections:
  World Frame/RConn1 -- Transform Sensor2/LConn1 -- Transform Sensor1/LConn1
  Transform Sensor2/RConn4 -- PS-Simulink Converter7/LConn1 -- PS-Simulink Converter3/LConn1
  Transform Sensor1/RConn4 -- PS-Simulink Converter6/LConn1 -- PS-Simulink Converter2/LConn1
  PS-Simulink Converter5/LConn1 -- Transform Sensor2/RConn3
  PS-Simulink Converter4/LConn1 -- Transform Sensor1/RConn3
  Transform Sensor2/RConn2 -- PS-Simulink Converter1/LConn1
  PS-Simulink Converter/LConn1 -- Transform Sensor1/RConn2
  Transform Sensor1/RConn1 -- Con1_up/RConn1
  Con2_down/RConn1 -- Transform Sensor2/RConn1

== system Crane_rigid/Controllers/controller 20 ==
  vd_x : Inport
  vd_y : Inport  Port=2
  v_x : Inport  Port=3
  v_y : Inport  Port=4
  ad_x : Inport  Port=5
  ad_y : Inport  Port=6
  theta_x : Inport  Port=7
  theta_y : Inport  Port=8
  theta_dot_x : Inport  Port=9
  theta_dot_y : Inport  Port=10
  Controllers : MATLAB Function  TreatAsAtomicUnit=on
  cont_param_20 : Constant  Value="1e3*[1.7494    3.4491         0    1.9071    2.9117 ]"
  h : Constant  Value=h
  total_mass : Constant  Value=total_mass
  F_x : Outport
  F_y : Outport  Port=2
  wires:
  Controllers/1(F_x) -> F_x/1
  Controllers/2(F_y) -> F_y/1
  v_x/1 -> Controllers/3(v_x)
  v_y/1 -> Controllers/4(v_y)
  vd_y/1 -> Controllers/2(vd_y)
  vd_x/1 -> Controllers/1(vd_x)
  ad_x/1 -> Controllers/5(ad_x)
  ad_y/1 -> Controllers/6(ad_y)
  theta_x/1 -> Controllers/7(theta_x)
  theta_y/1 -> Controllers/8(theta_y)
  theta_dot_x/1 -> Controllers/9(theta_dot_x)
  theta_dot_y/1 -> Controllers/10(theta_dot_y)
  h/1 -> Controllers/11(h)
  total_mass/1 -> Controllers/13(total_mass)
  cont_param_20/1 -> Controllers/12(cont_param_20)

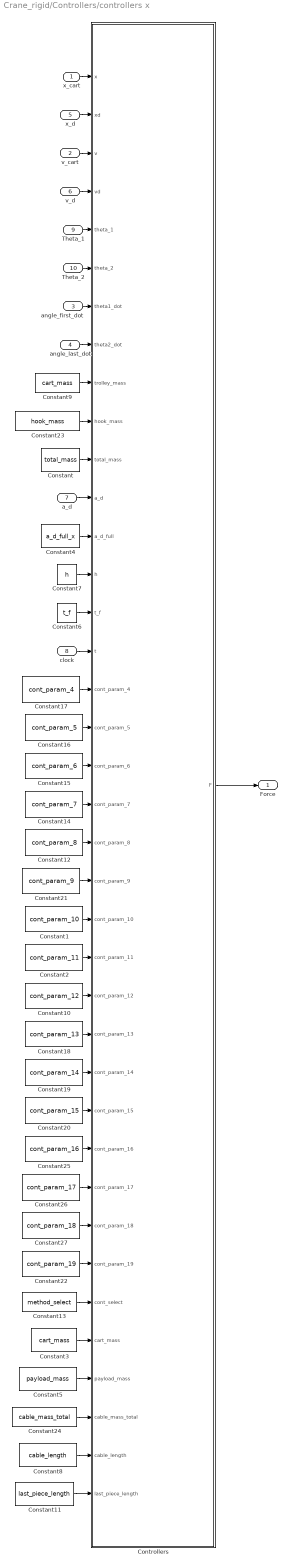
== system Crane_rigid/Controllers/controllers x ==
  x_cart : Inport
  v_cart : Inport  Port=2
  angle_first_dot : Inport  Port=3
  angle_last_dot : Inport  Port=4
  x_d : Inport  Port=5
  v_d : Inport  Port=6
  a_d : Inport  Port=7
  clock : Inport  Port=8
  Theta_1 : Inport  Port=9
  Theta_2 : Inport  Port=10
  Constant : Constant  Value=total_mass
  Constant1 : Constant  Value=cont_param_10
  Constant10 : Constant  Value=cont_param_12
  Constant11 : Constant  Value=last_piece_length
  Constant12 : Constant  Value=cont_param_8
  Constant13 : Constant  Value=method_select
  Constant14 : Constant  Value=cont_param_7
  Constant15 : Constant  Value=cont_param_6
  Constant16 : Constant  Value=cont_param_5
  Constant17 : Constant  Value=cont_param_4
  Constant18 : Constant  Value=cont_param_13
  Constant19 : Constant  Value=cont_param_14
  Constant2 : Constant  Value=cont_param_11
  Constant20 : Constant  Value=cont_param_15
  Constant21 : Constant  Value=cont_param_9
  Constant22 : Constant  Value=cont_param_19
  Constant23 : Constant  Value=hook_mass
  Constant24 : Constant  Value=cable_mass_total
  Constant25 : Constant  Value=cont_param_16
  Constant26 : Constant  Value=cont_param_17
  Constant27 : Constant  Value=cont_param_18
  Constant3 : Constant  Value=cart_mass
  Constant4 : Constant  Value=a_d_full_x
  Constant5 : Constant  Value=payload_mass
  Constant6 : Constant  Value=t_f
  Constant7 : Constant  Value=h
  Constant8 : Constant  Value=cable_length
  Constant9 : Constant  Value=cart_mass
  Controllers : MATLAB Function  TreatAsAtomicUnit=on
  Force : Outport
  wires:
  Constant/1 -> Controllers/11(total_mass)
  Constant13/1 -> Controllers/33(cont_select)
  Constant21/1 -> Controllers/22(cont_param_9)
  Constant12/1 -> Controllers/21(cont_param_8)
  Constant15/1 -> Controllers/19(cont_param_6)
  Constant16/1 -> Controllers/18(cont_param_5)
  Constant17/1 -> Controllers/17(cont_param_4)
  Controllers/1(F) -> Force/1
  v_d/1 -> Controllers/4(vd)
  a_d/1 -> Controllers/12(a_d)
  clock/1 -> Controllers/16(t)
  Theta_1/1 -> Controllers/5(theta_1)
  Theta_2/1 -> Controllers/6(theta_2)
  x_d/1 -> Controllers/2(xd)
  v_cart/1 -> Controllers/3(v)
  x_cart/1 -> Controllers/1(x)
  Constant24/1 -> Controllers/36(cable_mass_total)
  Constant9/1 -> Controllers/9(trolley_mass)
  Constant4/1 -> Controllers/13(a_d_full)
  Constant7/1 -> Controllers/14(h)
  Constant6/1 -> Controllers/15(t_f)
  Constant23/1 -> Controllers/10(hook_mass)
  angle_first_dot/1 -> Controllers/7(theta1_dot)
  angle_last_dot/1 -> Controllers/8(theta2_dot)
  Constant14/1 -> Controllers/20(cont_param_7)
  Constant1/1 -> Controllers/23(cont_param_10)
  Constant2/1 -> Controllers/24(cont_param_11)
  Constant3/1 -> Controllers/34(cart_mass)
  Constant5/1 -> Controllers/35(payload_mass)
  Constant8/1 -> Controllers/37(cable_length)
  Constant11/1 -> Controllers/38(last_piece_length)
  Constant10/1 -> Controllers/25(cont_param_12)
  Constant18/1 -> Controllers/26(cont_param_13)
  Constant19/1 -> Controllers/27(cont_param_14)
  Constant20/1 -> Controllers/28(cont_param_15)
  Constant25/1 -> Controllers/29(cont_param_16)
  Constant26/1 -> Controllers/30(cont_param_17)
  Constant27/1 -> Controllers/31(cont_param_18)
  Constant22/1 -> Controllers/32(cont_param_19)

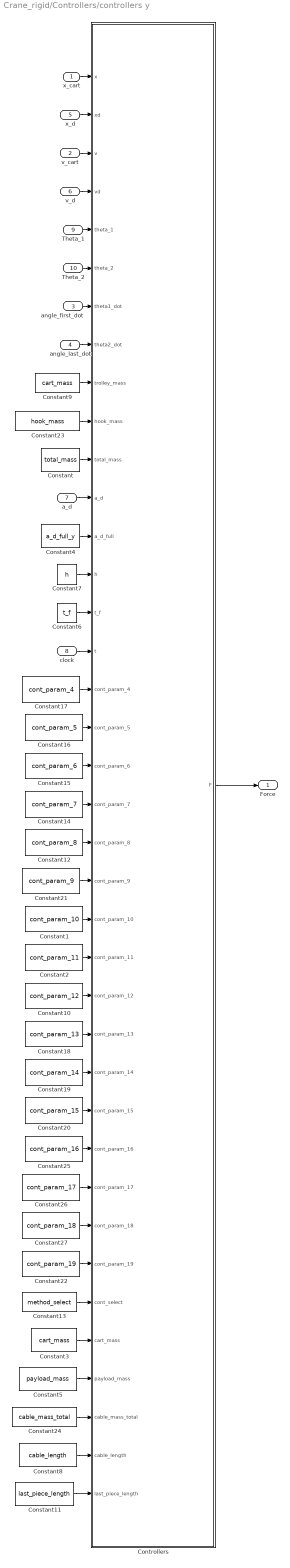
== system Crane_rigid/Controllers/controllers y ==
  x_cart : Inport
  v_cart : Inport  Port=2
  angle_first_dot : Inport  Port=3
  angle_last_dot : Inport  Port=4
  x_d : Inport  Port=5
  v_d : Inport  Port=6
  a_d : Inport  Port=7
  clock : Inport  Port=8
  Theta_1 : Inport  Port=9
  Theta_2 : Inport  Port=10
  Constant : Constant  Value=total_mass
  Constant1 : Constant  Value=cont_param_10
  Constant10 : Constant  Value=cont_param_12
  Constant11 : Constant  Value=last_piece_length
  Constant12 : Constant  Value=cont_param_8
  Constant13 : Constant  Value=method_select
  Constant14 : Constant  Value=cont_param_7
  Constant15 : Constant  Value=cont_param_6
  Constant16 : Constant  Value=cont_param_5
  Constant17 : Constant  Value=cont_param_4
  Constant18 : Constant  Value=cont_param_13
  Constant19 : Constant  Value=cont_param_14
  Constant2 : Constant  Value=cont_param_11
  Constant20 : Constant  Value=cont_param_15
  Constant21 : Constant  Value=cont_param_9
  Constant22 : Constant  Value=cont_param_19
  Constant23 : Constant  Value=hook_mass
  Constant24 : Constant  Value=cable_mass_total
  Constant25 : Constant  Value=cont_param_16
  Constant26 : Constant  Value=cont_param_17
  Constant27 : Constant  Value=cont_param_18
  Constant3 : Constant  Value=cart_mass
  Constant4 : Constant  Value=a_d_full_y
  Constant5 : Constant  Value=payload_mass
  Constant6 : Constant  Value=t_f
  Constant7 : Constant  Value=h
  Constant8 : Constant  Value=cable_length
  Constant9 : Constant  Value=cart_mass
  Controllers : MATLAB Function  TreatAsAtomicUnit=on
  Force : Outport
  wires:
  Constant/1 -> Controllers/11(total_mass)
  Constant13/1 -> Controllers/33(cont_select)
  Constant21/1 -> Controllers/22(cont_param_9)
  Constant12/1 -> Controllers/21(cont_param_8)
  Constant15/1 -> Controllers/19(cont_param_6)
  Constant16/1 -> Controllers/18(cont_param_5)
  Constant17/1 -> Controllers/17(cont_param_4)
  Controllers/1(F) -> Force/1
  v_d/1 -> Controllers/4(vd)
  a_d/1 -> Controllers/12(a_d)
  clock/1 -> Controllers/16(t)
  Theta_1/1 -> Controllers/5(theta_1)
  Theta_2/1 -> Controllers/6(theta_2)
  x_d/1 -> Controllers/2(xd)
  v_cart/1 -> Controllers/3(v)
  x_cart/1 -> Controllers/1(x)
  Constant24/1 -> Controllers/36(cable_mass_total)
  Constant9/1 -> Controllers/9(trolley_mass)
  Constant4/1 -> Controllers/13(a_d_full)
  Constant7/1 -> Controllers/14(h)
  Constant6/1 -> Controllers/15(t_f)
  Constant23/1 -> Controllers/10(hook_mass)
  angle_first_dot/1 -> Controllers/7(theta1_dot)
  angle_last_dot/1 -> Controllers/8(theta2_dot)
  Constant14/1 -> Controllers/20(cont_param_7)
  Constant1/1 -> Controllers/23(cont_param_10)
  Constant2/1 -> Controllers/24(cont_param_11)
  Constant3/1 -> Controllers/34(cart_mass)
  Constant5/1 -> Controllers/35(payload_mass)
  Constant8/1 -> Controllers/37(cable_length)
  Constant11/1 -> Controllers/38(last_piece_length)
  Constant10/1 -> Controllers/25(cont_param_12)
  Constant18/1 -> Controllers/26(cont_param_13)
  Constant19/1 -> Controllers/27(cont_param_14)
  Constant20/1 -> Controllers/28(cont_param_15)
  Constant25/1 -> Controllers/29(cont_param_16)
  Constant26/1 -> Controllers/30(cont_param_17)
  Constant27/1 -> Controllers/31(cont_param_18)
  Constant22/1 -> Controllers/32(cont_param_19)

== matlab function Crane_rigid/Controllers/controllers y/Controllers ==
  data: x input; xd input; v input; vd input; theta_1 input; theta_2 input; theta1_dot input; theta2_dot input; trolley_mass input; hook_mass input; total_mass input; a_d input; a_d_full input; h input; t_f input; t input; cont_param_4 input; cont_param_5 input; cont_param_6 input; cont_param_7 input; cont_param_8 input; cont_param_9 input; cont_param_10 input; cont_param_11 input; cont_param_12 input; cont_param_13 input; cont_param_14 input; cont_param_15 input; cont_param_16 input; cont_param_17 input; cont_param_18 input; cont_param_19 input; cont_select input; cart_mass input; payload_mass input; cable_mass_total input; F output; cable_length input; last_piece_length input
function F  = Control_select(x,xd,v,vd,theta_1,theta_2,theta1_dot,theta2_dot,trolley_mass,hook_mass,total_mass,a_d,a_d_full,h,t_f,t,cont_param_4,cont_param_5,cont_param_6,cont_param_7,cont_param_8,cont_param_9,cont_param_10,cont_param_11,cont_param_12,cont_param_13,cont_param_14,cont_param_15,cont_param_16,cont_param_17,cont_param_18,cont_param_19,cont_select,cart_mass,payload_mass,cable_mass_total,cable_length,last_piece_length)


    F = Controllers(x,xd,v,vd,theta_1,theta_2,theta1_dot,theta2_dot,trolley_mass,hook_mass,total_mass,a_d,a_d_full,h,t_f,t,cont_param_4,cont_param_5,cont_param_6,cont_param_7,cont_param_8,cont_param_9,cont_param_10,cont_param_11,cont_param_12,cont_param_13,cont_param_14,cont_param_15,cont_param_16,cont_param_17,cont_param_18,cont_param_19,cont_select,cart_mass,payload_mass,cable_mass_total,cable_length,last_piece_length);
                 
    if isnan(F)
        F=0;
    end
    
    
end

== matlab function Crane_rigid/trajectory generator/traj1_y ==
  data: t input; x_d output; v_d output; a_d output; traj_number input; sin_traj_w input; sin_traj_A input
function [x_d,v_d,a_d] = traj_gen(t,traj_number,sin_traj_w,sin_traj_A)
     [x_d,v_d,a_d] = trajectory(t,traj_number,sin_traj_w,sin_traj_A);
end

== matlab function Crane_rigid/trajectory generator/traj_x ==
  data: t input; x_d output; v_d output; a_d output; traj_number input; sin_traj_w input; sin_traj_A input
function [x_d,v_d,a_d] = traj_gen(t,traj_number,sin_traj_w,sin_traj_A)
     [x_d,v_d,a_d] = trajectory(t,traj_number,sin_traj_w,sin_traj_A);
end

== matlab function Crane_rigid/Controllers/controller 20/Controllers ==
  settings: updateMethod=DISCRETE
  data: vd_x input; vd_y input; v_x input; v_y input; ad_x input; ad_y input; theta_x input; theta_y input; theta_dot_x input; theta_dot_y input; h input; cont_param_20 input; total_mass input; F_x output; F_y output
function [F_x,F_y] = Control_select(vd_x,vd_y, v_x,v_y,ad_x,ad_y, theta_x, theta_y, theta_dot_x,theta_dot_y,h,cont_param_20,total_mass)
    [F_x,F_y] = control_20_coupling_tracking_3d_first(vd_x,vd_y, v_x,v_y,ad_x,ad_y, theta_x, theta_y, theta_dot_x,theta_dot_y,h,cont_param_20,total_mass);

== matlab function Crane_rigid/Controllers/controllers x/Controllers ==
  settings: updateMethod=DISCRETE
  data: x input; xd input; v input; vd input; theta_1 input; theta_2 input; theta1_dot input; theta2_dot input; trolley_mass input; hook_mass input; total_mass input; a_d input; a_d_full input; h input; t_f input; t input; cont_param_4 input; cont_param_5 input; cont_param_6 input; cont_param_7 input; cont_param_8 input; cont_param_9 input; cont_param_10 input; cont_param_11 input; cont_param_12 input; cont_param_13 input; cont_param_14 input; cont_param_15 input; cont_param_16 input; cont_param_17 input; cont_param_18 input; cont_param_19 input; cont_select input; cart_mass input; payload_mass input; cable_mass_total input; F output; cable_length input; last_piece_length input
function F  = Control_select(x,xd,v,vd,theta_1,theta_2,theta1_dot,theta2_dot,trolley_mass,hook_mass,total_mass,a_d,a_d_full,h,t_f,t,cont_param_4,cont_param_5,cont_param_6,cont_param_7,cont_param_8,cont_param_9,cont_param_10,cont_param_11,cont_param_12,cont_param_13,cont_param_14,cont_param_15,cont_param_16,cont_param_17,cont_param_18,cont_param_19,cont_select,cart_mass,payload_mass,cable_mass_total,cable_length,last_piece_length)

    F = Controllers(x,xd,v,vd,theta_1,theta_2,theta1_dot,theta2_dot,trolley_mass,hook_mass,total_mass,a_d,a_d_full,h,t_f,t,cont_param_4,cont_param_5,cont_param_6,cont_param_7,cont_param_8,cont_param_9,cont_param_10,cont_param_11,cont_param_12,cont_param_13,cont_param_14,cont_param_15,cont_param_16,cont_param_17,cont_param_18,cont_param_19,cont_select,cart_mass,payload_mass,cable_mass_total,cable_length,last_piece_length);
                 
    if isnan(F)
        F=0;
    end
    
    
end
